simulink model "bateau"  (R2025a)
settings: Solver=VariableStepAuto  StartTime=0.0  StopTime=20  RelTol=1e-3
values from neighbouring files (symbols this model uses):
  A_pa = [0 1 ... (first row only)    [bateau_data.m]
  b = 1e9    (= 1000000000)    [bateau_data.m]    (also in chariot_data.m; porte_avion.m)
  B_pa = [0 ... (first row only)    [bateau_data.m]
  c = 0.4e9    (= 400000000)    [bateau_data.m]    (also in chariot_data.m; porte_avion.m)
  C_pa = [1 0]    [bateau_data.m]
  d = 500e6    (= 500000000)    [bateau_data.m]    (also in chariot_data.m; porte_avion.m)
  D_pa = 0    [bateau_data.m]
  f = 60    [bateau_data.m]    (also in chariot_data.m; porte_avion.m)
settings Model: Creator=vikfo  LastModifiedBy=vikfo

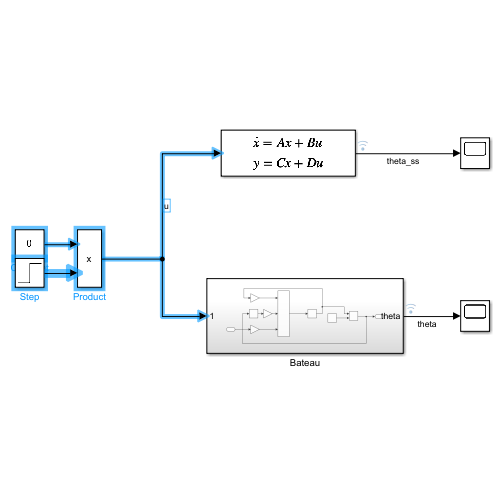
[thumbnail: Simulink's stored preview of the top-level diagram]
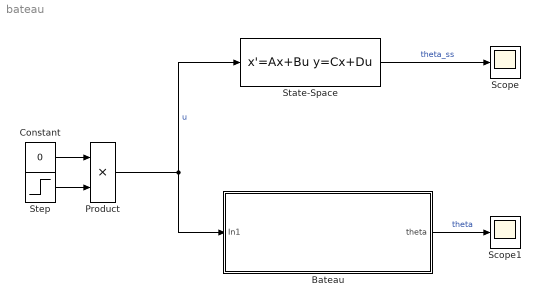
== system bateau ==
  Bateau : Subsystem
  Constant : Constant  Value=0
  Product : Product
  Scope : Scope
      settings: ActiveDisplayYMinimum=-1  ActiveDisplayYMaximum=1
  Scope1 : Scope
      settings: ActiveDisplayYMinimum=-0.17835109837862997  ActiveDisplayYMaximum=0.36888263910760255
  State-Space : StateSpace  A=A_pa  B=B_pa  C=C_pa  D=D_pa  InitialCondition=[pi/10; 0]  ParameterTunability=Unconstrained
  Step : Step  SampleTime=0
  wires:
  State-Space/1 -> Scope/1  "theta_ss"
  Constant/1 -> Product/1
  Step/1 -> Product/2
  Product/1 -> Bateau/1(In1), State-Space/1  "u"
  Bateau/1(theta) -> Scope1/1  "theta"

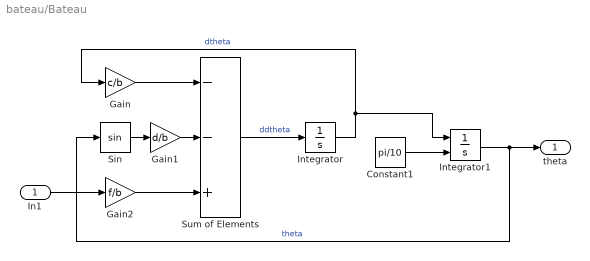
== system bateau/Bateau ==
  In1 : Inport
  Constant1 : Constant  Value=pi/10
  Gain : Gain  Gain=c/b
  Gain1 : Gain  Gain=d/b
  Gain2 : Gain  Gain=f/b
  Integrator : Integrator
  Integrator1 : Integrator  InitialConditionSource=external
  Sin : Trigonometry
  Sum of Elements : Sum  Inputs=--+
  theta : Outport
  wires:
  Integrator/1 -> Gain/1, Integrator1/1  "dtheta"
  In1/1 -> Gain2/1
  Sum of Elements/1 -> Integrator/1  "ddtheta"
  Gain/1 -> Sum of Elements/1
  Gain2/1 -> Sum of Elements/3
  Integrator1/1 -> Sin/1, theta/1  "theta"
  Gain1/1 -> Sum of Elements/2
  Constant1/1 -> Integrator1/2
  Sin/1 -> Gain1/1
